simulink model "sl_ztorque"  (R2015b)
settings: Solver=ode45  StartTime=0.0  StopTime=5  RelTol=1e-3
libraries: roblocks x2
settings Model: ExtModeTrigMode=oneshot  ExtModeArmWhenConnect=off  Creator=pic  LastModifiedBy=corkep
settings DataIOCC: LimitDataPoints=off  SaveFormat=Array  SignalLoggingSaveFormat=ModelDataLogs  SignalLogging=off  ReturnWorkspaceOutputs=on
settings OptimizationCC: BlockReduction=off  BooleanDataType=off  ExpressionDepthLimit=2147483647  InitFltsAndDblsToZero=on
settings DebuggingCC: SaveWithParameterizedLinksMsg=none  UnderspecifiedInitializationDetection=Classic  MergeDetectMultiDrivingBlocksExec=none  SignalResolutionControl=TryResolveAllWithWarning  MultiTaskDSMMsg=warning  MultiTaskCondExecSysMsg=none  FcnCallInpInsideContextMsg=UseLocalSettings  StateNameClashWarn=warning
settings HardwareCC: ProdBitPerPointer=32  ProdLargestAtomicFloat=None  ProdIntDivRoundTo=Undefined  ProdEndianess=Unspecified  ProdWordSize=32  ProdHWDeviceType=32-bit Generic  TargetUnknown=on
settings GRTTargetCC: ModelReferenceCompliant=off  ParMdlRefBuildCompliant=off  CompOptLevelCompliant=off  GeneratePreprocessorConditionals=Disable all  CombineOutputUpdateFcns=off  MatFileLogging=off  GRTInterface=on
settings ConfigComp: CovModelRefEnable=Off  CovSFcnEnable=off

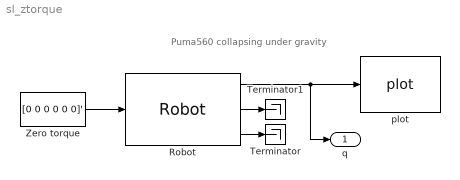
== system sl_ztorque ==
  note: Puma560 collapsing under gravity
  Robot : roblocks/Arm/Robot  robot=p560.nofriction  q0=[0 0 0 0 0 0]
  Terminator : Terminator
  Terminator1 : Terminator
  Zero torque : Constant  Value=[0 0 0 0 0 0]'
  plot : roblocks/Arm/plot  robot=p560  fps=25  holdplot=on
  q : Outport
  wires:
  Zero torque/1 -> Robot/1
  Robot/1 -> plot/1, q/1
  Robot/3 -> Terminator/1
  Robot/2 -> Terminator1/1
